simulink library "ILCPurePursuitCtrl_cl"  (R2018b)
settings: Solver=VariableStepAuto  StartTime=0.0  StopTime=10.0  RelTol=1e-3
values from neighbouring files (symbols this model uses):
  numberOfLaps_none = 5    [ILCPurePursuitCtrl_cl_init.m]
undefined symbols (not defined in the file or in its folder): deltauStar, linPlntDisc
libraries: simulink x1, headingSetpointNumerical_cl x1
settings Model: Creator=mcobb  LastModifiedBy=mitch
settings DebuggingCC: LibraryContextMissingDiagnostic=none
settings SFSimCC: SimUseLocalCustomCode=off
settings RTWCC: RTWUseLocalCustomCode=off

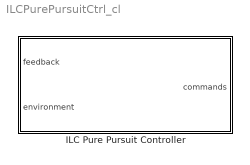
== system ILCPurePursuitCtrl_cl ==
  ILC Pure Pursuit Controller : Subsystem  VariantControl=VSS_PUREPURSUIT_CTRL

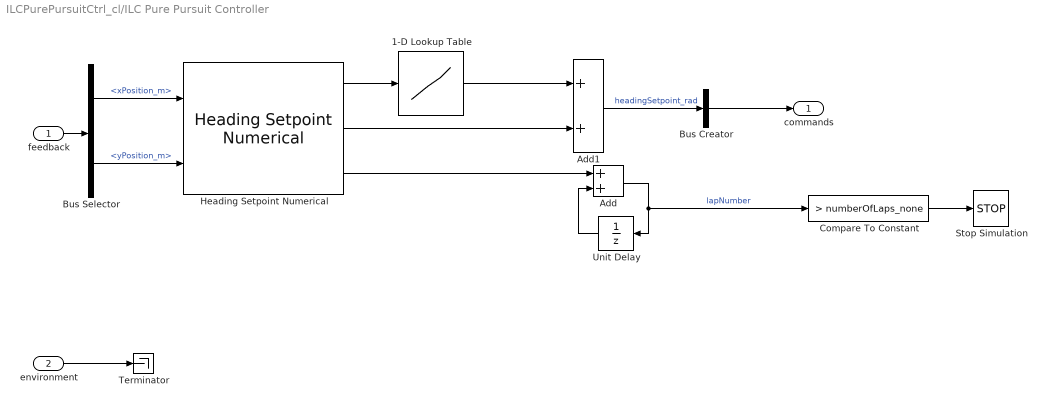
== system ILCPurePursuitCtrl_cl/ILC Pure Pursuit Controller ==
  feedback : Inport
  environment : Inport  Port=2
  1-D Lookup Table : Lookup_n-D  NumberOfTableDimensions=1  BreakpointsForDimension1=linPlntDisc.ctrlInput.Time  Table=deltauStar  ExtrapMethod=Clip  UseLastTableValue=on  InternalRulePriority=Speed  RndMeth=Simplest  InputSameDT=on
  Add : Sum
  Add1 : Sum
  Bus Creator : BusCreator  Inputs=1
  Bus Selector : BusSelector  OutputSignals=xPosition_m,yPosition_m
  Compare To Constant : simulink/Logic and Bit Operations/Compare To Constant  relop=>  const=numberOfLaps_none  OutDataTypeStr=boolean
  Heading Setpoint Numerical : headingSetpointNumerical_cl/Heading Setpoint Numerical  SystemSampleTime=-1
  Stop Simulation : Stop
  Terminator : Terminator
  Unit Delay : UnitDelay  InitialCondition=1  SampleTime=-1
  commands : Outport
  wires:
  feedback/1 -> Bus Selector/1
  Bus Selector/1 -> Heading Setpoint Numerical/1  "<xPosition_m>"
  Bus Selector/2 -> Heading Setpoint Numerical/2  "<yPosition_m>"
  environment/1 -> Terminator/1
  Heading Setpoint Numerical/2 -> Add1/2
  Bus Creator/1 -> commands/1
  Compare To Constant/1 -> Stop Simulation/1
  Heading Setpoint Numerical/1 -> 1-D Lookup Table/1
  1-D Lookup Table/1 -> Add1/1
  Add1/1 -> Bus Creator/1  "headingSetpoint_rad"
  Heading Setpoint Numerical/3 -> Add/1
  Unit Delay/1 -> Add/2
  Add/1 -> Compare To Constant/1, Unit Delay/1  "lapNumber"
